simulink model "LUT_kidney_25"  (R2023b)
settings: Solver=FixedStepAuto  StartTime=0  StopTime=10.1  FixedStep=Timegap  RelTol=1e-3
model workspace (MAT data in the model file):
  T1_input = 1.34
(part 3 of 3)

== system LUT_kidney_25/If Action Subsystem6/If Action Subsystem2/If Action Subsystem9/If Action Subsystem11 ==
  In1 : Inport
  Action Port : ActionPort  ActionPortLabel=elseif( u1 >= 1.905)
  LUT 1.91RR : Lookup_n-D  NumberOfTableDimensions=1  BreakpointsForDimension1=[427.7417;526.5879;622.5189;718.2471;813.5689;908.5848;1003.378;1098.008;1192.516;1286.933;1381.278;1475.567;1569.812;1664.022;1758.202;1852.359;1946.495]  Table=[400;500;600;700;800;900;1000;1100;1200;1300;1400;1500;1600;1700;1800;1900;2000]  InternalRulePriority=Speed  RndMeth=Simplest
  Out1 : Outport
  wires:
  In1/1 -> LUT 1.91RR/1
  LUT 1.91RR/1 -> Out1/1

== system LUT_kidney_25/If Action Subsystem6/If Action Subsystem2/If Action Subsystem9/If Action Subsystem2 ==
  In1 : Inport
  Action Port : ActionPort  ActionPortLabel=else
  LUT 1.90RR : Lookup_n-D  NumberOfTableDimensions=1  BreakpointsForDimension1=[427.7886;526.638;622.5756;718.3151;813.6521;908.6864;1003.501;1098.153;1192.686;1287.128;1381.499;1475.815;1570.088;1664.325;1758.534;1852.72;1946.885]  Table=[400;500;600;700;800;900;1000;1100;1200;1300;1400;1500;1600;1700;1800;1900;2000]  InternalRulePriority=Speed  RndMeth=Simplest
  Out1 : Outport
  wires:
  In1/1 -> LUT 1.90RR/1
  LUT 1.90RR/1 -> Out1/1

== system LUT_kidney_25/If Action Subsystem6/If Action Subsystem2/If Action Subsystem9/If Action Subsystem3 ==
  In1 : Inport
  Action Port : ActionPort  ActionPortLabel=elseif( u1 >= 1.925)
  LUT 1.93RR : Lookup_n-D  NumberOfTableDimensions=1  BreakpointsForDimension1=[427.6492;526.4895;622.4082;718.1147;813.4071;908.3872;1003.14;1097.725;1192.186;1286.553;1380.846;1475.083;1569.274;1663.428;1757.553;1851.653;1945.733]  Table=[400;500;600;700;800;900;1000;1100;1200;1300;1400;1500;1600;1700;1800;1900;2000]  InternalRulePriority=Speed  RndMeth=Simplest
  Out1 : Outport
  wires:
  In1/1 -> LUT 1.93RR/1
  LUT 1.93RR/1 -> Out1/1

== system LUT_kidney_25/If Action Subsystem6/If Action Subsystem2/If Action Subsystem9/If Action Subsystem4 ==
  In1 : Inport
  Action Port : ActionPort  ActionPortLabel=elseif( u1 >= 1.935)
  LUT 1.94RR : Lookup_n-D  NumberOfTableDimensions=1  BreakpointsForDimension1=[427.6036;526.4412;622.3541;718.0503;813.3284;908.2911;1003.024;1097.588;1192.026;1286.368;1380.636;1474.847;1569.011;1663.139;1757.236;1851.308;1945.36]  Table=[400;500;600;700;800;900;1000;1100;1200;1300;1400;1500;1600;1700;1800;1900;2000]  InternalRulePriority=Speed  RndMeth=Simplest
  Out1 : Outport
  wires:
  In1/1 -> LUT 1.94RR/1
  LUT 1.94RR/1 -> Out1/1

== system LUT_kidney_25/If Action Subsystem6/If Action Subsystem2/If Action Subsystem9/If Action Subsystem5 ==
  In1 : Inport
  Action Port : ActionPort  ActionPortLabel=elseif( u1 >= 1.955)
  LUT 1.96RR : Lookup_n-D  NumberOfTableDimensions=1  BreakpointsForDimension1=[427.5135;526.3463;622.2484;717.9249;813.1755;908.1045;1002.799;1097.32;1191.713;1286.007;1380.226;1474.386;1568.498;1662.572;1756.616;1850.634;1944.63]  Table=[400;500;600;700;800;900;1000;1100;1200;1300;1400;1500;1600;1700;1800;1900;2000]  InternalRulePriority=Speed  RndMeth=Simplest
  Out1 : Outport
  wires:
  In1/1 -> LUT 1.96RR/1
  LUT 1.96RR/1 -> Out1/1

== system LUT_kidney_25/If Action Subsystem6/If Action Subsystem2/If Action Subsystem9/If Action Subsystem6 ==
  In1 : Inport
  Action Port : ActionPort  ActionPortLabel=elseif( u1 >= 1.945)
  LUT 1.95RR : Lookup_n-D  NumberOfTableDimensions=1  BreakpointsForDimension1=[427.5584;526.3934;622.3008;717.987;813.2513;908.1969;1002.91;1097.453;1191.868;1286.186;1380.429;1474.614;1568.752;1662.853;1756.923;1850.968;1944.992]  Table=[400;500;600;700;800;900;1000;1100;1200;1300;1400;1500;1600;1700;1800;1900;2000]  InternalRulePriority=Speed  RndMeth=Simplest
  Out1 : Outport
  wires:
  In1/1 -> LUT 1.95RR/1
  LUT 1.95RR/1 -> Out1/1

== system LUT_kidney_25/If Action Subsystem6/If Action Subsystem2/If Action Subsystem9/If Action Subsystem7 ==
  In1 : Inport
  Action Port : ActionPort  ActionPortLabel=elseif( u1 >= 1.965)
  LUT 1.97RR : Lookup_n-D  NumberOfTableDimensions=1  BreakpointsForDimension1=[427.469;526.2997;622.1967;717.8638;813.1012;908.0139;1002.689;1097.19;1191.56;1285.832;1380.026;1474.161;1568.248;1662.296;1756.313;1850.304;1944.273]  Table=[400;500;600;700;800;900;1000;1100;1200;1300;1400;1500;1600;1700;1800;1900;2000]  InternalRulePriority=Speed  RndMeth=Simplest
  Out1 : Outport
  wires:
  In1/1 -> LUT 1.97RR/1
  LUT 1.97RR/1 -> Out1/1

== system LUT_kidney_25/If Action Subsystem6/If Action Subsystem2/If Action Subsystem9/If Action Subsystem8 ==
  In1 : Inport
  Action Port : ActionPort  ActionPortLabel=elseif( u1 >= 1.975)
  LUT 1.98RR : Lookup_n-D  NumberOfTableDimensions=1  BreakpointsForDimension1=[427.425;526.2536;622.1459;717.8039;813.0283;907.9249;1002.582;1097.062;1191.411;1285.659;1379.83;1473.94;1568.001;1662.024;1756.015;1849.979;1943.922]  Table=[400;500;600;700;800;900;1000;1100;1200;1300;1400;1500;1600;1700;1800;1900;2000]  InternalRulePriority=Speed  RndMeth=Simplest
  Out1 : Outport
  wires:
  In1/1 -> LUT 1.98RR/1
  LUT 1.98RR/1 -> Out1/1

== system LUT_kidney_25/If Action Subsystem6/If Action Subsystem2/If Action Subsystem9/If Action Subsystem9 ==
  In1 : Inport
  Action Port : ActionPort  ActionPortLabel=elseif(u1 >= 1.985)
  LUT 1.99RR : Lookup_n-D  NumberOfTableDimensions=1  BreakpointsForDimension1=[427.3813;526.2081;622.0958;717.7449;812.9568;907.8376;1002.476;1096.937;1191.264;1285.489;1379.636;1473.722;1567.759;1661.756;1755.721;1849.659;1943.576]  Table=[400;500;600;700;800;900;1000;1100;1200;1300;1400;1500;1600;1700;1800;1900;2000]  InternalRulePriority=Speed  RndMeth=Simplest
  Out1 : Outport
  wires:
  In1/1 -> LUT 1.99RR/1
  LUT 1.99RR/1 -> Out1/1

== system LUT_kidney_25/If Action Subsystem6/If Action Subsystem3/If Action Subsystem5/If Action Subsystem1 ==
  In1 : Inport
  Action Port : ActionPort  ActionPortLabel=elseif( u1 >= 0.615)
  LUT 0.62RR : Lookup_n-D  NumberOfTableDimensions=1  BreakpointsForDimension1=[446.0088;557.1267;665.4287;774.0652;882.6285;991.1427;1099.656;1208.215;1316.862;1425.625;1534.479;1642.545;1754.018;1863.53;1973.555;2083.978;2194.803]  Table=[400;500;600;700;800;900;1000;1100;1200;1300;1400;1500;1600;1700;1800;1900;2000]  InternalRulePriority=Speed  RndMeth=Simplest
  Out1 : Outport
  wires:
  In1/1 -> LUT 0.62RR/1
  LUT 0.62RR/1 -> Out1/1

== system LUT_kidney_25/If Action Subsystem6/If Action Subsystem3/If Action Subsystem5/If Action Subsystem10 ==
  In1 : Inport
  Action Port : ActionPort  ActionPortLabel=elseif( u1 >= 0.605)
  LUT 0.61RR : Lookup_n-D  NumberOfTableDimensions=1  BreakpointsForDimension1=[446.4753;558.3907;667.3641;776.6183;885.7663;994.8484;1103.924;1213.051;1322.277;1431.633;1541.077;1654.628;1761.975;1872.286;1983.112;2094.382;2206.109]  Table=[400;500;600;700;800;900;1000;1100;1200;1300;1400;1500;1600;1700;1800;1900;2000]  InternalRulePriority=Speed  RndMeth=Simplest
  Out1 : Outport
  wires:
  In1/1 -> LUT 0.61RR/1
  LUT 0.61RR/1 -> Out1/1

== system LUT_kidney_25/If Action Subsystem6/If Action Subsystem3/If Action Subsystem5/If Action Subsystem2 ==
  In1 : Inport
  Action Port : ActionPort  ActionPortLabel=else
  LUT 0.6RR : Lookup_n-D  NumberOfTableDimensions=1  BreakpointsForDimension1=[446.9422;559.7362;669.4438;779.3696;889.1513;998.8481;1108.534;1218.275;1328.13;1438.132;1548.209;1661.173;1770.629;1881.8;1993.509;2105.718;2218.447]  Table=[400;500;600;700;800;900;1000;1100;1200;1300;1400;1500;1600;1700;1800;1900;2000]  InternalRulePriority=Speed  RndMeth=Simplest
  Out1 : Outport
  wires:
  In1/1 -> LUT 0.6RR/1
  LUT 0.6RR/1 -> Out1/1

== system LUT_kidney_25/If Action Subsystem6/If Action Subsystem3/If Action Subsystem5/If Action Subsystem3 ==
  In1 : Inport
  Action Port : ActionPort  ActionPortLabel=elseif( u1 >= 0.625)
  LUT 0.63RR : Lookup_n-D  NumberOfTableDimensions=1  BreakpointsForDimension1=[445.5457;555.9382;663.6243;771.6913;879.7135;987.7014;1095.693;1203.727;1311.838;1420.053;1528.359;1636.296;1746.694;1855.446;1964.742;2074.398;2184.408]  Table=[400;500;600;700;800;900;1000;1100;1200;1300;1400;1500;1600;1700;1800;1900;2000]  InternalRulePriority=Speed  RndMeth=Simplest
  Out1 : Outport
  wires:
  In1/1 -> LUT 0.63RR/1
  LUT 0.63RR/1 -> Out1/1

== system LUT_kidney_25/If Action Subsystem6/If Action Subsystem3/If Action Subsystem5/If Action Subsystem4 ==
  In1 : Inport
  Action Port : ActionPort  ActionPortLabel=elseif( u1 >= 0.635)
  LUT 0.64RR : Lookup_n-D  NumberOfTableDimensions=1  BreakpointsForDimension1=[445.0885;554.8196;661.9394;769.4796;876.9996;984.4983;1092.004;1199.55;1307.166;1414.873;1522.668;1630.294;1739.964;1847.962;1956.591;2065.548;2174.82]  Table=[400;500;600;700;800;900;1000;1100;1200;1300;1400;1500;1600;1700;1800;1900;2000]  InternalRulePriority=Speed  RndMeth=Simplest
  Out1 : Outport
  wires:
  In1/1 -> LUT 0.64RR/1
  LUT 0.64RR/1 -> Out1/1

== system LUT_kidney_25/If Action Subsystem6/If Action Subsystem3/If Action Subsystem5/If Action Subsystem5 ==
  In1 : Inport
  Action Port : ActionPort  ActionPortLabel=elseif( u1 >= 0.655)
  LUT 0.66RR : Lookup_n-D  NumberOfTableDimensions=1  BreakpointsForDimension1=[444.1991;552.7715;658.8868;765.484;872.1006;978.7169;1085.348;1192.014;1298.736;1405.532;1512.404;1619.262;1728.471;1834.549;1941.993;2049.729;2157.715]  Table=[400;500;600;700;800;900;1000;1100;1200;1300;1400;1500;1600;1700;1800;1900;2000]  InternalRulePriority=Speed  RndMeth=Simplest
  Out1 : Outport
  wires:
  In1/1 -> LUT 0.66RR/1
  LUT 0.66RR/1 -> Out1/1

== system LUT_kidney_25/If Action Subsystem6/If Action Subsystem3/If Action Subsystem5/If Action Subsystem6 ==
  In1 : Inport
  Action Port : ActionPort  ActionPortLabel=elseif( u1 >= 0.645)
  LUT 0.65RR : Lookup_n-D  NumberOfTableDimensions=1  BreakpointsForDimension1=[444.6392;553.7656;660.3634;767.415;874.4676;981.5103;1088.564;1195.655;1302.809;1410.045;1517.362;1624.613;1733.838;1841.014;1949.028;2057.349;2165.948]  Table=[400;500;600;700;800;900;1000;1100;1200;1300;1400;1500;1600;1700;1800;1900;2000]  InternalRulePriority=Speed  RndMeth=Simplest
  Out1 : Outport
  wires:
  In1/1 -> LUT 0.65RR/1
  LUT 0.65RR/1 -> Out1/1

== system LUT_kidney_25/If Action Subsystem6/If Action Subsystem3/If Action Subsystem5/If Action Subsystem7 ==
  In1 : Inport
  Action Port : ActionPort  ActionPortLabel=elseif( u1 >= 0.665)
  LUT 0.67RR : Lookup_n-D  NumberOfTableDimensions=1  BreakpointsForDimension1=[443.7692;551.833;657.5011;763.6748;869.8833;976.1;1082.334;1188.602;1294.92;1401.305;1507.76;1614.228;1724.482;1828.519;1935.429;2042.628;2150.051]  Table=[400;500;600;700;800;900;1000;1100;1200;1300;1400;1500;1600;1700;1800;1900;2000]  InternalRulePriority=Speed  RndMeth=Simplest
  Out1 : Outport
  wires:
  In1/1 -> LUT 0.67RR/1
  LUT 0.67RR/1 -> Out1/1

== system LUT_kidney_25/If Action Subsystem6/If Action Subsystem3/If Action Subsystem5/If Action Subsystem8 ==
  In1 : Inport
  Action Port : ActionPort  ActionPortLabel=elseif(u1 >= 0.675)
  LUT 0.68RR : Lookup_n-D  NumberOfTableDimensions=1  BreakpointsForDimension1=[443.3505;550.9459;656.1987;761.9764;867.8022;973.6433;1079.504;1185.397;1291.337;1397.336;1503.399;1609.49;1714.737;1822.886;1929.289;2035.992;2142.897]  Table=[400;500;600;700;800;900;1000;1100;1200;1300;1400;1500;1600;1700;1800;1900;2000]  InternalRulePriority=Speed  RndMeth=Simplest
  Out1 : Outport
  wires:
  In1/1 -> LUT 0.68RR/1
  LUT 0.68RR/1 -> Out1/1

== system LUT_kidney_25/If Action Subsystem6/If Action Subsystem3/If Action Subsystem5/If Action Subsystem9 ==
  In1 : Inport
  Action Port : ActionPort  ActionPortLabel=if(u1 >= 0.685)
  LUT 0.69RR : Lookup_n-D  NumberOfTableDimensions=1  BreakpointsForDimension1=[442.9433;550.1066;654.9725;760.3793;865.8452;971.3325;1076.841;1182.382;1287.964;1393.6;1499.295;1605.025;1710.391;1817.622;1923.532;2029.773;2136.201]  Table=[400;500;600;700;800;900;1000;1100;1200;1300;1400;1500;1600;1700;1800;1900;2000]  InternalRulePriority=Speed  RndMeth=Simplest
  Out1 : Outport
  wires:
  In1/1 -> LUT 0.69RR/1
  LUT 0.69RR/1 -> Out1/1

== system LUT_kidney_25/If Action Subsystem6/If Action Subsystem3/If Action Subsystem6/If Action Subsystem1 ==
  In1 : Inport
  Action Port : ActionPort  ActionPortLabel=elseif( u1 >= 0.515)
  LUT 0.52RR : Lookup_n-D  NumberOfTableDimensions=1  BreakpointsForDimension1=[449.9366;574.3493;693.4557;811.7788;929.3907;1046.66;1163.89;1281.332;1399.203;1517.741;1636.994;1757.112;1878.385;2000.885;2124.742;2250.088;2377.058]  Table=[400;500;600;700;800;900;1000;1100;1200;1300;1400;1500;1600;1700;1800;1900;2000]  InternalRulePriority=Speed  RndMeth=Simplest
  Out1 : Outport
  wires:
  In1/1 -> LUT 0.52RR/1
  LUT 0.52RR/1 -> Out1/1

== system LUT_kidney_25/If Action Subsystem6/If Action Subsystem3/If Action Subsystem6/If Action Subsystem10 ==
  In1 : Inport
  Action Port : ActionPort  ActionPortLabel=elseif( u1 >= 0.505)
  LUT 0.51RR : Lookup_n-D  NumberOfTableDimensions=1  BreakpointsForDimension1=[450.047;576.7952;697.7542;817.7093;936.8348;1055.571;1174.275;1293.244;1412.754;1533.272;1653.559;1775.841;1899.306;2024.17;2150.605;2278.77;2408.832]  Table=[400;500;600;700;800;900;1000;1100;1200;1300;1400;1500;1600;1700;1800;1900;2000]  InternalRulePriority=Speed  RndMeth=Simplest
  Out1 : Outport
  wires:
  In1/1 -> LUT 0.51RR/1
  LUT 0.51RR/1 -> Out1/1

== system LUT_kidney_25/If Action Subsystem6/If Action Subsystem3/If Action Subsystem6/If Action Subsystem2 ==
  In1 : Inport
  Action Port : ActionPort  ActionPortLabel=else
  LUT 0.50RR : Lookup_n-D  NumberOfTableDimensions=1  BreakpointsForDimension1=[450.0331;579.414;702.4543;824.239;945.0609;1065.444;1185.809;1306.511;1427.913;1548.382;1672.144;1796.814;1922.778;2050.353;2179.751;2311.167;2444.809]  Table=[400;500;600;700;800;900;1000;1100;1200;1300;1400;1500;1600;1700;1800;1900;2000]  InternalRulePriority=Speed  RndMeth=Simplest
  Out1 : Outport
  wires:
  In1/1 -> LUT 0.50RR/1
  LUT 0.50RR/1 -> Out1/1

== system LUT_kidney_25/If Action Subsystem6/If Action Subsystem3/If Action Subsystem6/If Action Subsystem3 ==
  In1 : Inport
  Action Port : ActionPort  ActionPortLabel=elseif( u1 >= 0.525)
  LUT 0.53RR : Lookup_n-D  NumberOfTableDimensions=1  BreakpointsForDimension1=[449.7287;572.0652;689.5181;806.3806;922.6372;1038.595;1154.512;1270.599;1387.034;1503.951;1622.252;1740.331;1859.671;1980.099;2101.705;2224.596;2348.882]  Table=[400;500;600;700;800;900;1000;1100;1200;1300;1400;1500;1600;1700;1800;1900;2000]  InternalRulePriority=Speed  RndMeth=Simplest
  Out1 : Outport
  wires:
  In1/1 -> LUT 0.53RR/1
  LUT 0.53RR/1 -> Out1/1

== system LUT_kidney_25/If Action Subsystem6/If Action Subsystem3/If Action Subsystem6/If Action Subsystem4 ==
  In1 : Inport
  Action Port : ActionPort  ActionPortLabel=elseif( u1 >= 0.535)
  LUT 0.54RR : Lookup_n-D  NumberOfTableDimensions=1  BreakpointsForDimension1=[449.445;569.9316;685.9048;801.4562;916.495;1031.276;1146.015;1260.895;1376.062;1491.602;1609.232;1725.247;1842.871;1961.476;2081.108;2201.852;2323.799]  Table=[400;500;600;700;800;900;1000;1100;1200;1300;1400;1500;1600;1700;1800;1900;2000]  InternalRulePriority=Speed  RndMeth=Simplest
  Out1 : Outport
  wires:
  In1/1 -> LUT 0.54RR/1
  LUT 0.54RR/1 -> Out1/1

== system LUT_kidney_25/If Action Subsystem6/If Action Subsystem3/If Action Subsystem6/If Action Subsystem5 ==
  In1 : Inport
  Action Port : ActionPort  ActionPortLabel=elseif( u1 >= 0.555)
  LUT 0.56RR : Lookup_n-D  NumberOfTableDimensions=1  BreakpointsForDimension1=[448.7176;566.0743;679.525;792.8289;905.7757;1018.534;1131.26;1244.083;1357.109;1470.391;1588.548;1699.359;1814.057;1929.62;2045.977;2163.173;2281.272]  Table=[400;500;600;700;800;900;1000;1100;1200;1300;1400;1500;1600;1700;1800;1900;2000]  InternalRulePriority=Speed  RndMeth=Simplest
  Out1 : Outport
  wires:
  In1/1 -> LUT 0.56RR/1
  LUT 0.56RR/1 -> Out1/1

== system LUT_kidney_25/If Action Subsystem6/If Action Subsystem3/If Action Subsystem6/If Action Subsystem6 ==
  In1 : Inport
  Action Port : ActionPort  ActionPortLabel=elseif( u1 >= 0.545)
  LUT 0.55RR : Lookup_n-D  NumberOfTableDimensions=1  BreakpointsForDimension1=[449.1031;567.9381;682.5835;796.954;910.8946;1024.614;1138.295;1252.093;1366.13;1480.472;1597.966;1711.648;1827.737;1944.731;2062.624;2181.483;2301.382]  Table=[400;500;600;700;800;900;1000;1100;1200;1300;1400;1500;1600;1700;1800;1900;2000]  InternalRulePriority=Speed  RndMeth=Simplest
  Out1 : Outport
  wires:
  In1/1 -> LUT 0.55RR/1
  LUT 0.55RR/1 -> Out1/1

== system LUT_kidney_25/If Action Subsystem6/If Action Subsystem3/If Action Subsystem6/If Action Subsystem7 ==
  In1 : Inport
  Action Port : ActionPort  ActionPortLabel=elseif( u1 >= 0.565)
  LUT 0.57RR : Lookup_n-D  NumberOfTableDimensions=1  BreakpointsForDimension1=[448.3001;564.3309;676.7036;789.041;901.0853;1012.972;1124.83;1236.772;1348.887;1461.222;1573.48;1688.236;1801.65;1915.936;2030.929;2146.655;2263.164]  Table=[400;500;600;700;800;900;1000;1100;1200;1300;1400;1500;1600;1700;1800;1900;2000]  InternalRulePriority=Speed  RndMeth=Simplest
  Out1 : Outport
  wires:
  In1/1 -> LUT 0.57RR/1
  LUT 0.57RR/1 -> Out1/1

== system LUT_kidney_25/If Action Subsystem6/If Action Subsystem3/If Action Subsystem6/If Action Subsystem8 ==
  In1 : Inport
  Action Port : ActionPort  ActionPortLabel=elseif(u1 >= 0.575)
  LUT 0.58RR : Lookup_n-D  NumberOfTableDimensions=1  BreakpointsForDimension1=[447.8602;562.6989;674.0962;785.5551;896.7773;1007.869;1118.938;1230.079;1341.369;1452.85;1564.332;1678.173;1790.362;1903.503;2017.279;2131.698;2246.799]  Table=[400;500;600;700;800;900;1000;1100;1200;1300;1400;1500;1600;1700;1800;1900;2000]  InternalRulePriority=Speed  RndMeth=Simplest
  Out1 : Outport
  wires:
  In1/1 -> LUT 0.58RR/1
  LUT 0.58RR/1 -> Out1/1

== system LUT_kidney_25/If Action Subsystem6/If Action Subsystem3/If Action Subsystem6/If Action Subsystem9 ==
  In1 : Inport
  Action Port : ActionPort  ActionPortLabel=if(u1 >= 0.585)
  LUT 0.59RR : Lookup_n-D  NumberOfTableDimensions=1  BreakpointsForDimension1=[447.4055;561.1699;671.6824;782.3404;892.8112;1003.175;1113.523;1223.933;1334.473;1445.181;1555.937;1669.126;1780.059;1892.168;2004.855;2118.108;2231.956]  Table=[400;500;600;700;800;900;1000;1100;1200;1300;1400;1500;1600;1700;1800;1900;2000]  InternalRulePriority=Speed  RndMeth=Simplest
  Out1 : Outport
  wires:
  In1/1 -> LUT 0.59RR/1
  LUT 0.59RR/1 -> Out1/1

== system LUT_kidney_25/If Action Subsystem6/If Action Subsystem3/If Action Subsystem7/If Action Subsystem1 ==
  In1 : Inport
  Action Port : ActionPort  ActionPortLabel=elseif( u1 >= 0.715)
  LUT 0.72RR : Lookup_n-D  NumberOfTableDimensions=1  BreakpointsForDimension1=[441.7934;547.8423;651.6923;756.1135;860.6165;965.1533;1069.716;1174.307;1278.931;1383.594;1488.302;1593.047;1697.757;1804.231;1908.209;2013.235;2118.425]  Table=[400;500;600;700;800;900;1000;1100;1200;1300;1400;1500;1600;1700;1800;1900;2000]  InternalRulePriority=Speed  RndMeth=Simplest
  Out1 : Outport
  wires:
  In1/1 -> LUT 0.72RR/1
  LUT 0.72RR/1 -> Out1/1

== system LUT_kidney_25/If Action Subsystem6/If Action Subsystem3/If Action Subsystem7/If Action Subsystem10 ==
  In1 : Inport
  Action Port : ActionPort  ActionPortLabel=elseif( u1 >= 0.705)
  LUT 0.71RR : Lookup_n-D  NumberOfTableDimensions=1  BreakpointsForDimension1=[442.1646;548.5578;652.7247;757.4553;862.2616;967.0984;1071.96;1176.85;1281.777;1386.747;1491.766;1596.823;1701.8;1808.188;1913.022;2018.429;2124.003]  Table=[400;500;600;700;800;900;1000;1100;1200;1300;1400;1500;1600;1700;1800;1900;2000]  InternalRulePriority=Speed  RndMeth=Simplest
  Out1 : Outport
  wires:
  In1/1 -> LUT 0.71RR/1
  LUT 0.71RR/1 -> Out1/1

== system LUT_kidney_25/If Action Subsystem6/If Action Subsystem3/If Action Subsystem7/If Action Subsystem2 ==
  In1 : Inport
  Action Port : ActionPort  ActionPortLabel=else
  LUT 0.70RR : Lookup_n-D  NumberOfTableDimensions=1  BreakpointsForDimension1=[442.5479;549.3116;653.8164;758.8749;864.0016;969.1547;1074.331;1179.538;1284.783;1390.077;1495.424;1600.809;1706.024;1812.713;1918.12;2023.931;2129.916]  Table=[400;500;600;700;800;900;1000;1100;1200;1300;1400;1500;1600;1700;1800;1900;2000]  InternalRulePriority=Speed  RndMeth=Simplest
  Out1 : Outport
  wires:
  In1/1 -> LUT 0.70RR/1
  LUT 0.70RR/1 -> Out1/1

== system LUT_kidney_25/If Action Subsystem6/If Action Subsystem3/If Action Subsystem7/If Action Subsystem3 ==
  In1 : Inport
  Action Port : ActionPort  ActionPortLabel=elseif( u1 >= 0.725)
  LUT 0.73RR : Lookup_n-D  NumberOfTableDimensions=1  BreakpointsForDimension1=[441.4341;547.1625;650.7145;754.8434;859.0586;963.3103;1067.589;1171.894;1276.23;1380.603;1485.015;1589.463;1693.9;1801.782;1903.659;2008.322;2113.152]  Table=[400;500;600;700;800;900;1000;1100;1200;1300;1400;1500;1600;1700;1800;1900;2000]  InternalRulePriority=Speed  RndMeth=Simplest
  Out1 : Outport
  wires:
  In1/1 -> LUT 0.73RR/1
  LUT 0.73RR/1 -> Out1/1

== system LUT_kidney_25/If Action Subsystem6/If Action Subsystem3/If Action Subsystem7/If Action Subsystem4 ==
  In1 : Inport
  Action Port : ActionPort  ActionPortLabel=elseif( u1 >= 0.735)
  LUT 0.74RR : Lookup_n-D  NumberOfTableDimensions=1  BreakpointsForDimension1=[441.0865;546.5158;649.7873;753.6391;857.5808;961.5611;1065.568;1169.602;1273.664;1377.759;1481.89;1586.055;1690.223;1793.713;1899.353;2003.664;2108.155]  Table=[400;500;600;700;800;900;1000;1100;1200;1300;1400;1500;1600;1700;1800;1900;2000]  InternalRulePriority=Speed  RndMeth=Simplest
  Out1 : Outport
  wires:
  In1/1 -> LUT 0.74RR/1
  LUT 0.74RR/1 -> Out1/1

== system LUT_kidney_25/If Action Subsystem6/If Action Subsystem3/If Action Subsystem7/If Action Subsystem5 ==
  In1 : Inport
  Action Port : ActionPort  ActionPortLabel=elseif( u1 >= 0.755)
  LUT 0.76RR : Lookup_n-D  NumberOfTableDimensions=1  BreakpointsForDimension1=[440.4259;545.3131;648.0692;751.408;854.841;958.3148;1061.816;1165.341;1268.892;1372.469;1476.077;1579.713;1683.365;1786.88;1891.432;1995.029;2098.898]  Table=[400;500;600;700;800;900;1000;1100;1200;1300;1400;1500;1600;1700;1800;1900;2000]  InternalRulePriority=Speed  RndMeth=Simplest
  Out1 : Outport
  wires:
  In1/1 -> LUT 0.76RR/1
  LUT 0.76RR/1 -> Out1/1

== system LUT_kidney_25/If Action Subsystem6/If Action Subsystem3/If Action Subsystem7/If Action Subsystem6 ==
  In1 : Inport
  Action Port : ActionPort  ActionPortLabel=elseif( u1 >= 0.745)
  LUT 0.75RR : Lookup_n-D  NumberOfTableDimensions=1  BreakpointsForDimension1=[440.7506;545.9;648.9066;752.4955;856.1769;959.8981;1063.647;1167.42;1271.221;1375.052;1478.915;1582.809;1686.715;1790.339;1895.277;1999.239;2103.411]  Table=[400;500;600;700;800;900;1000;1100;1200;1300;1400;1500;1600;1700;1800;1900;2000]  InternalRulePriority=Speed  RndMeth=Simplest
  Out1 : Outport
  wires:
  In1/1 -> LUT 0.75RR/1
  LUT 0.75RR/1 -> Out1/1

== system LUT_kidney_25/If Action Subsystem6/If Action Subsystem3/If Action Subsystem7/If Action Subsystem7 ==
  In1 : Inport
  Action Port : ActionPort  ActionPortLabel=elseif( u1 >= 0.765)
  LUT 0.77RR : Lookup_n-D  NumberOfTableDimensions=1  BreakpointsForDimension1=[440.1121;544.753;647.2718;750.3725;853.5681;956.805;1060.069;1163.356;1266.667;1370.003;1473.366;1576.755;1680.161;1783.497;1887.852;1991.015;2094.596]  Table=[400;500;600;700;800;900;1000;1100;1200;1300;1400;1500;1600;1700;1800;1900;2000]  InternalRulePriority=Speed  RndMeth=Simplest
  Out1 : Outport
  wires:
  In1/1 -> LUT 0.77RR/1
  LUT 0.77RR/1 -> Out1/1

== system LUT_kidney_25/If Action Subsystem6/If Action Subsystem3/If Action Subsystem7/If Action Subsystem8 ==
  In1 : Inport
  Action Port : ActionPort  ActionPortLabel=elseif(u1 >= 0.775)
  LUT 0.78RR : Lookup_n-D  NumberOfTableDimensions=1  BreakpointsForDimension1=[439.809;544.2181;646.5115;749.385;852.3535;955.3633;1058.4;1161.459;1264.54;1367.643;1470.771;1573.924;1677.094;1780.228;1884.75;1987.184;2090.488]  Table=[400;500;600;700;800;900;1000;1100;1200;1300;1400;1500;1600;1700;1800;1900;2000]  InternalRulePriority=Speed  RndMeth=Simplest
  Out1 : Outport
  wires:
  In1/1 -> LUT 0.78RR/1
  LUT 0.78RR/1 -> Out1/1

== system LUT_kidney_25/If Action Subsystem6/If Action Subsystem3/If Action Subsystem7/If Action Subsystem9 ==
  In1 : Inport
  Action Port : ActionPort  ActionPortLabel=if(u1 >= 0.785)
  LUT 0.79RR : Lookup_n-D  NumberOfTableDimensions=1  BreakpointsForDimension1=[439.516;543.7067;645.7858;748.4421;851.1929;953.9848;1056.803;1159.642;1262.502;1365.383;1468.286;1571.211;1674.154;1777.079;1878.322;1983.523;2086.56]  Table=[400;500;600;700;800;900;1000;1100;1200;1300;1400;1500;1600;1700;1800;1900;2000]  InternalRulePriority=Speed  RndMeth=Simplest
  Out1 : Outport
  wires:
  In1/1 -> LUT 0.79RR/1
  LUT 0.79RR/1 -> Out1/1

== system LUT_kidney_25/If Action Subsystem6/If Action Subsystem3/If Action Subsystem8/If Action Subsystem1 ==
  In1 : Inport
  Action Port : ActionPort  ActionPortLabel=elseif( u1 >= 0.815)
  LUT 0.82RR : Lookup_n-D  NumberOfTableDimensions=1  BreakpointsForDimension1=[438.695;542.2988;643.7929;745.8509;847.999;950.1853;1052.395;1154.623;1256.868;1359.129;1461.407;1563.701;1666.01;1768.323;1870.532;1973.499;2075.719]  Table=[400;500;600;700;800;900;1000;1100;1200;1300;1400;1500;1600;1700;1800;1900;2000]  InternalRulePriority=Speed  RndMeth=Simplest
  Out1 : Outport
  wires:
  In1/1 -> LUT 0.82RR/1
  LUT 0.82RR/1 -> Out1/1

== system LUT_kidney_25/If Action Subsystem6/If Action Subsystem3/If Action Subsystem8/If Action Subsystem10 ==
  In1 : Inport
  Action Port : ActionPort  ActionPortLabel=elseif( u1 >= 0.805)
  LUT 0.81RR : Lookup_n-D  NumberOfTableDimensions=1  BreakpointsForDimension1=[438.9595;542.7484;644.4286;746.6778;849.019;951.3997;1053.805;1156.229;1258.672;1361.132;1463.61;1566.107;1668.62;1771.132;1873.44;1976.68;2079.187]  Table=[400;500;600;700;800;900;1000;1100;1200;1300;1400;1500;1600;1700;1800;1900;2000]  InternalRulePriority=Speed  RndMeth=Simplest
  Out1 : Outport
  wires:
  In1/1 -> LUT 0.81RR/1
  LUT 0.81RR/1 -> Out1/1

== system LUT_kidney_25/If Action Subsystem6/If Action Subsystem3/If Action Subsystem8/If Action Subsystem2 ==
  In1 : Inport
  Action Port : ActionPort  ActionPortLabel=else
  LUT 0.80RR : Lookup_n-D  NumberOfTableDimensions=1  BreakpointsForDimension1=[439.233;543.2172;645.0922;747.5406;850.0826;952.6649;1055.273;1157.901;1260.548;1363.215;1465.901;1568.608;1671.332;1774.049;1876.284;1980.023;2082.797]  Table=[400;500;600;700;800;900;1000;1100;1200;1300;1400;1500;1600;1700;1800;1900;2000]  InternalRulePriority=Speed  RndMeth=Simplest
  Out1 : Outport
  wires:
  In1/1 -> LUT 0.80RR/1
  LUT 0.80RR/1 -> Out1/1

== system LUT_kidney_25/If Action Subsystem6/If Action Subsystem3/If Action Subsystem8/If Action Subsystem3 ==
  In1 : Inport
  Action Port : ActionPort  ActionPortLabel=elseif( u1 >= 0.825)
  LUT 0.83RR : Lookup_n-D  NumberOfTableDimensions=1  BreakpointsForDimension1=[438.4393;541.8673;643.1833;745.0577;847.0197;949.0185;1051.04;1153.078;1255.132;1357.201;1459.285;1561.384;1663.497;1765.615;1867.676;1970.523;2072.386]  Table=[400;500;600;700;800;900;1000;1100;1200;1300;1400;1500;1600;1700;1800;1900;2000]  InternalRulePriority=Speed  RndMeth=Simplest
  Out1 : Outport
  wires:
  In1/1 -> LUT 0.83RR/1
  LUT 0.83RR/1 -> Out1/1

== system LUT_kidney_25/If Action Subsystem6/If Action Subsystem3/If Action Subsystem8/If Action Subsystem4 ==
  In1 : Inport
  Action Port : ActionPort  ActionPortLabel=elseif( u1 >= 0.835)
  LUT 0.84RR : Lookup_n-D  NumberOfTableDimensions=1  BreakpointsForDimension1=[438.192;541.4527;642.5982;744.2958;846.0784;947.8962;1049.735;1151.59;1253.46;1355.343;1457.24;1559.15;1661.073;1763.003;1864.899;1968.021;2069.177]  Table=[400;500;600;700;800;900;1000;1100;1200;1300;1400;1500;1600;1700;1800;1900;2000]  InternalRulePriority=Speed  RndMeth=Simplest
  Out1 : Outport
  wires:
  In1/1 -> LUT 0.84RR/1
  LUT 0.84RR/1 -> Out1/1

== system LUT_kidney_25/If Action Subsystem6/If Action Subsystem3/If Action Subsystem8/If Action Subsystem5 ==
  In1 : Inport
  Action Port : ActionPort  ActionPortLabel=elseif( u1 >= 0.855)
  LUT 0.86RR : Lookup_n-D  NumberOfTableDimensions=1  BreakpointsForDimension1=[437.7153;540.6706;641.4953;742.8585;844.3006;945.7742;1047.266;1148.772;1250.29;1351.819;1453.36;1554.911;1656.473;1758.043;1859.601;1960.824;2063.112]  Table=[400;500;600;700;800;900;1000;1100;1200;1300;1400;1500;1600;1700;1800;1900;2000]  InternalRulePriority=Speed  RndMeth=Simplest
  Out1 : Outport
  wires:
  In1/1 -> LUT 0.86RR/1
  LUT 0.86RR/1 -> Out1/1

== system LUT_kidney_25/If Action Subsystem6/If Action Subsystem3/If Action Subsystem8/If Action Subsystem6 ==
  In1 : Inport
  Action Port : ActionPort  ActionPortLabel=elseif( u1 >= 0.845)
  LUT 0.85RR : Lookup_n-D  NumberOfTableDimensions=1  BreakpointsForDimension1=[437.9527;541.0541;642.036;743.5634;845.1728;946.8156;1048.478;1150.156;1251.847;1353.55;1455.266;1556.994;1658.734;1760.48;1862.208;1962.783;2066.087]  Table=[400;500;600;700;800;900;1000;1100;1200;1300;1400;1500;1600;1700;1800;1900;2000]  InternalRulePriority=Speed  RndMeth=Simplest
  Out1 : Outport
  wires:
  In1/1 -> LUT 0.85RR/1
  LUT 0.85RR/1 -> Out1/1

== system LUT_kidney_25/If Action Subsystem6/If Action Subsystem3/If Action Subsystem8/If Action Subsystem7 ==
  In1 : Inport
  Action Port : ActionPort  ActionPortLabel=elseif( u1 >= 0.865)
  LUT 0.87RR : Lookup_n-D  NumberOfTableDimensions=1  BreakpointsForDimension1=[437.4966;540.3011;640.9747;742.1796;843.4599;944.7696;1046.096;1147.436;1248.786;1350.146;1451.517;1552.897;1654.288;1755.685;1857.075;1958.316;2060.252]  Table=[400;500;600;700;800;900;1000;1100;1200;1300;1400;1500;1600;1700;1800;1900;2000]  InternalRulePriority=Speed  RndMeth=Simplest
  Out1 : Outport
  wires:
  In1/1 -> LUT 0.87RR/1
  LUT 0.87RR/1 -> Out1/1

== system LUT_kidney_25/If Action Subsystem6/If Action Subsystem3/If Action Subsystem8/If Action Subsystem8 ==
  In1 : Inport
  Action Port : ActionPort  ActionPortLabel=elseif(u1 >= 0.875)
  LUT 0.88RR : Lookup_n-D  NumberOfTableDimensions=1  BreakpointsForDimension1=[437.2791;539.945;640.4731;741.5251;842.6488;943.7996;1044.966;1146.144;1247.331;1348.528;1449.734;1550.949;1652.172;1753.402;1854.629;1955.775;2057.517]  Table=[400;500;600;700;800;900;1000;1100;1200;1300;1400;1500;1600;1700;1800;1900;2000]  InternalRulePriority=Speed  RndMeth=Simplest
  Out1 : Outport
  wires:
  In1/1 -> LUT 0.88RR/1
  LUT 0.88RR/1 -> Out1/1

== system LUT_kidney_25/If Action Subsystem6/If Action Subsystem3/If Action Subsystem8/If Action Subsystem9 ==
  In1 : Inport
  Action Port : ActionPort  ActionPortLabel=if(u1 >= 0.885)
  LUT 0.89RR : Lookup_n-D  NumberOfTableDimensions=1  BreakpointsForDimension1=[437.0683;539.6014;639.9894;740.8935;841.8655;942.8623;1043.873;1144.894;1245.924;1346.961;1448.007;1549.061;1650.123;1751.19;1852.257;1953.276;2054.963]  Table=[400;500;600;700;800;900;1000;1100;1200;1300;1400;1500;1600;1700;1800;1900;2000]  InternalRulePriority=Speed  RndMeth=Simplest
  Out1 : Outport
  wires:
  In1/1 -> LUT 0.89RR/1
  LUT 0.89RR/1 -> Out1/1

== system LUT_kidney_25/If Action Subsystem6/If Action Subsystem3/If Action Subsystem9/If Action Subsystem1 ==
  In1 : Inport
  Action Port : ActionPort  ActionPortLabel=elseif( u1 >= 0.915)
  LUT 0.92RR : Lookup_n-D  NumberOfTableDimensions=1  BreakpointsForDimension1=[436.4727;538.6392;638.6358;739.1242;839.6682;940.2294;1040.799;1141.376;1241.957;1342.545;1443.137;1543.735;1644.339;1744.947;1845.556;1946.153;2046.51]  Table=[400;500;600;700;800;900;1000;1100;1200;1300;1400;1500;1600;1700;1800;1900;2000]  InternalRulePriority=Speed  RndMeth=Simplest
  Out1 : Outport
  wires:
  In1/1 -> LUT 0.92RR/1
  LUT 0.92RR/1 -> Out1/1

== system LUT_kidney_25/If Action Subsystem6/If Action Subsystem3/If Action Subsystem9/If Action Subsystem10 ==
  In1 : Inport
  Action Port : ActionPort  ActionPortLabel=elseif( u1 >= 0.905)
  LUT 0.91RR : Lookup_n-D  NumberOfTableDimensions=1  BreakpointsForDimension1=[436.6654;538.9492;639.0717;739.6943;840.3766;941.0788;1041.792;1142.512;1243.239;1343.972;1444.712;1545.457;1646.209;1746.966;1847.724;1948.463;2048.467]  Table=[400;500;600;700;800;900;1000;1100;1200;1300;1400;1500;1600;1700;1800;1900;2000]  InternalRulePriority=Speed  RndMeth=Simplest
  Out1 : Outport
  wires:
  In1/1 -> LUT 0.91RR/1
  LUT 0.91RR/1 -> Out1/1

== system LUT_kidney_25/If Action Subsystem6/If Action Subsystem3/If Action Subsystem9/If Action Subsystem2 ==
  In1 : Inport
  Action Port : ActionPort  ActionPortLabel=else
  LUT 0.90RR : Lookup_n-D  NumberOfTableDimensions=1  BreakpointsForDimension1=[436.8638;539.2697;639.5226;740.2837;841.1086;941.956;1042.816;1143.684;1244.56;1345.444;1446.334;1547.232;1648.136;1749.046;1849.957;1950.837;2052.988]  Table=[400;500;600;700;800;900;1000;1100;1200;1300;1400;1500;1600;1700;1800;1900;2000]  InternalRulePriority=Speed  RndMeth=Simplest
  Out1 : Outport
  wires:
  In1/1 -> LUT 0.90RR/1
  LUT 0.90RR/1 -> Out1/1

== system LUT_kidney_25/If Action Subsystem6/If Action Subsystem3/If Action Subsystem9/If Action Subsystem3 ==
  In1 : Inport
  Action Port : ActionPort  ActionPortLabel=elseif( u1 >= 0.925)
  LUT 0.93RR : Lookup_n-D  NumberOfTableDimensions=1  BreakpointsForDimension1=[436.2855;538.3393;638.2142;738.5726;838.9821;939.4062;1039.837;1140.273;1240.714;1341.159;1441.609;1542.063;1642.522;1742.985;1843.45;1943.905;2044.245]  Table=[400;500;600;700;800;900;1000;1100;1200;1300;1400;1500;1600;1700;1800;1900;2000]  InternalRulePriority=Speed  RndMeth=Simplest
  Out1 : Outport
  wires:
  In1/1 -> LUT 0.93RR/1
  LUT 0.93RR/1 -> Out1/1

== system LUT_kidney_25/If Action Subsystem6/If Action Subsystem3/If Action Subsystem9/If Action Subsystem4 ==
  In1 : Inport
  Action Port : ActionPort  ActionPortLabel=elseif( u1 >= 0.935)
  LUT 0.94RR : Lookup_n-D  NumberOfTableDimensions=1  BreakpointsForDimension1=[436.1035;538.0489;637.806;738.0383;838.3172;938.608;1038.904;1139.203;1239.506;1339.813;1440.123;1540.438;1640.756;1741.078;1841.402;1941.719;2041.97]  Table=[400;500;600;700;800;900;1000;1100;1200;1300;1400;1500;1600;1700;1800;1900;2000]  InternalRulePriority=Speed  RndMeth=Simplest
  Out1 : Outport
  wires:
  In1/1 -> LUT 0.94RR/1
  LUT 0.94RR/1 -> Out1/1

== system LUT_kidney_25/If Action Subsystem6/If Action Subsystem3/If Action Subsystem9/If Action Subsystem5 ==
  In1 : Inport
  Action Port : ActionPort  ActionPortLabel=elseif( u1 >= 0.955)
  LUT 0.96RR : Lookup_n-D  NumberOfTableDimensions=1  BreakpointsForDimension1=[435.7542;537.4947;637.0276;737.0185;837.047;937.0817;1037.118;1137.155;1237.193;1337.233;1437.276;1537.321;1637.368;1737.419;1837.471;1937.519;2037.54]  Table=[400;500;600;700;800;900;1000;1100;1200;1300;1400;1500;1600;1700;1800;1900;2000]  InternalRulePriority=Speed  RndMeth=Simplest
  Out1 : Outport
  wires:
  In1/1 -> LUT 0.96RR/1
  LUT 0.96RR/1 -> Out1/1

== system LUT_kidney_25/If Action Subsystem6/If Action Subsystem3/If Action Subsystem9/If Action Subsystem6 ==
  In1 : Inport
  Action Port : ActionPort  ActionPortLabel=elseif( u1 >= 0.945)
  LUT 0.95RR : Lookup_n-D  NumberOfTableDimensions=1  BreakpointsForDimension1=[435.9265;537.7675;637.4107;737.5205;837.6725;937.8335;1037.998;1138.164;1238.333;1338.505;1438.68;1538.858;1639.039;1739.223;1839.409;1939.591;2039.731]  Table=[400;500;600;700;800;900;1000;1100;1200;1300;1400;1500;1600;1700;1800;1900;2000]  InternalRulePriority=Speed  RndMeth=Simplest
  Out1 : Outport
  wires:
  In1/1 -> LUT 0.95RR/1
  LUT 0.95RR/1 -> Out1/1

== system LUT_kidney_25/If Action Subsystem6/If Action Subsystem3/If Action Subsystem9/If Action Subsystem7 ==
  In1 : Inport
  Action Port : ActionPort  ActionPortLabel=elseif( u1 >= 0.965)
  LUT 0.97RR : Lookup_n-D  NumberOfTableDimensions=1  BreakpointsForDimension1=[435.5865;537.23;636.656;736.5314;836.4398;936.3515;1036.263;1136.173;1236.084;1335.996;1435.909;1535.825;1635.742;1735.662;1835.583;1935.501;2035.401]  Table=[400;500;600;700;800;900;1000;1100;1200;1300;1400;1500;1600;1700;1800;1900;2000]  InternalRulePriority=Speed  RndMeth=Simplest
  Out1 : Outport
  wires:
  In1/1 -> LUT 0.97RR/1
  LUT 0.97RR/1 -> Out1/1

== system LUT_kidney_25/If Action Subsystem6/If Action Subsystem3/If Action Subsystem9/If Action Subsystem8 ==
  In1 : Inport
  Action Port : ActionPort  ActionPortLabel=elseif(u1 >= 0.975)
  LUT 0.98RR : Lookup_n-D  NumberOfTableDimensions=1  BreakpointsForDimension1=[435.423;536.973;636.2954;736.0586;835.8501;935.6418;1035.431;1135.218;1235.005;1334.792;1434.579;1534.368;1634.159;1733.951;1833.744;1933.535;2033.313]  Table=[400;500;600;700;800;900;1000;1100;1200;1300;1400;1500;1600;1700;1800;1900;2000]  InternalRulePriority=Speed  RndMeth=Simplest
  Out1 : Outport
  wires:
  In1/1 -> LUT 0.98RR/1
  LUT 0.98RR/1 -> Out1/1

== system LUT_kidney_25/If Action Subsystem6/If Action Subsystem3/If Action Subsystem9/If Action Subsystem9 ==
  In1 : Inport
  Action Port : ActionPort  ActionPortLabel=if(u1 >= 0.985)
  LUT 0.99RR : Lookup_n-D  NumberOfTableDimensions=1  BreakpointsForDimension1=[435.2637;536.7234;635.9453;735.5994;835.277;934.9519;1034.622;1134.289;1233.954;1333.619;1433.284;1532.949;1632.616;1732.283;1831.952;1931.619;2031.276]  Table=[400;500;600;700;800;900;1000;1100;1200;1300;1400;1500;1600;1700;1800;1900;2000]  InternalRulePriority=Speed  RndMeth=Simplest
  Out1 : Outport
  wires:
  In1/1 -> LUT 0.99RR/1
  LUT 0.99RR/1 -> Out1/1
